simulink model "hybrid_aircraft"  (R2025b)
settings: Solver=ode4  StartTime=0.0  StopTime=1800  FixedStep=1  RelTol=1e-3
undefined symbols (not defined in the file): P_engine_max, P_motor_max
libraries: simulink x2

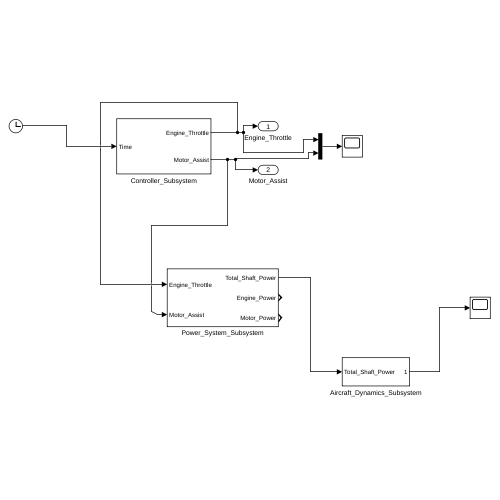
[thumbnail: Simulink's stored preview of the top-level diagram]
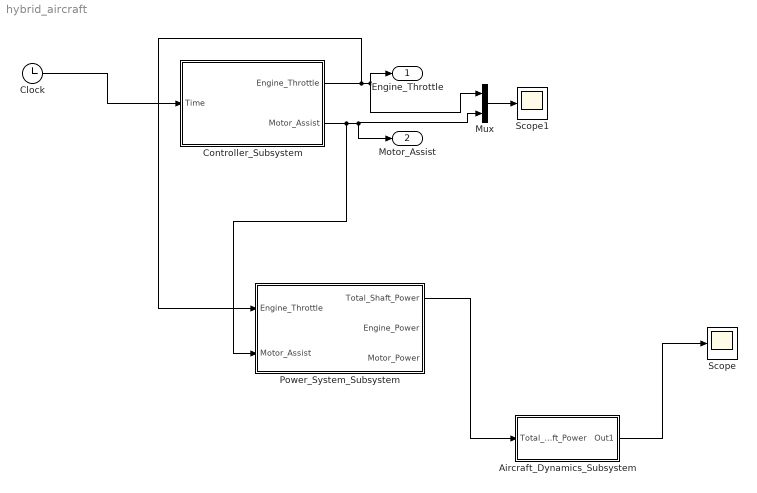
== system hybrid_aircraft ==
  Aircraft_Dynamics_Subsystem : Subsystem
  Clock : Clock
  Controller_Subsystem : Subsystem
  Mux : Mux  Inputs=2
  "Power_System_Subsystem " : Subsystem
  Scope : Scope
      settings: ActiveDisplayYMinimum=-317.16468253968424  ActiveDisplayYMaximum=2854.4821428571586
  Scope1 : Scope
      settings: ActiveDisplayYMinimum=-0.5175712749625333  ActiveDisplayYMaximum=1.2565171534864985
  Engine_Throttle : Outport
  Motor_Assist : Outport  Port=2
  wires:
  Clock/1 -> Controller_Subsystem/1(Time)
  Aircraft_Dynamics_Subsystem/1(Out1) -> Scope/1
  Controller_Subsystem/2(Motor_Assist) -> "Power_System_Subsystem "/2(Motor_Assist), Motor_Assist/1, Mux/2
  Controller_Subsystem/1(Engine_Throttle) -> "Power_System_Subsystem "/1(Engine_Throttle), Engine_Throttle/1, Mux/1
  Mux/1 -> Scope1/1
  "Power_System_Subsystem "/1(Total_Shaft_Power) -> Aircraft_Dynamics_Subsystem/1(Total_Shaft_Power)

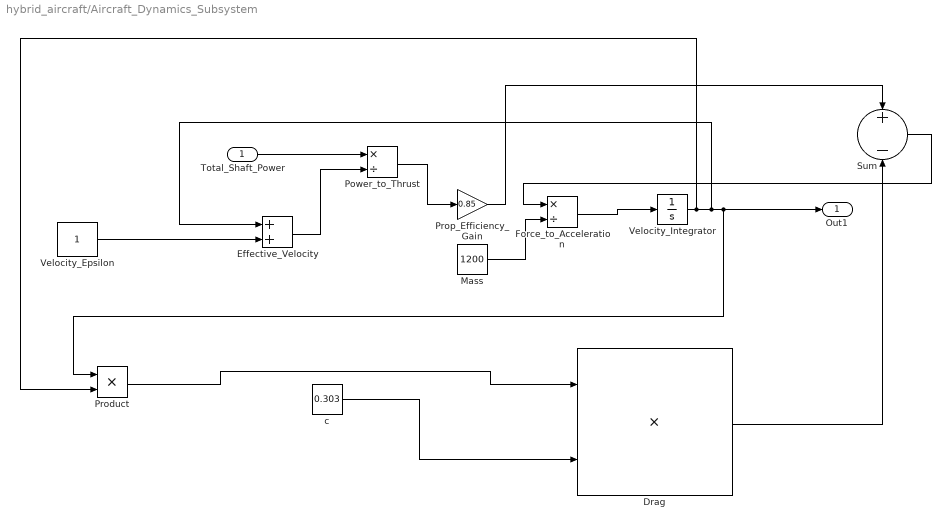
== system hybrid_aircraft/Aircraft_Dynamics_Subsystem ==
  Total_Shaft_Power : Inport
  Drag : Product
  Effective_Velocity : Sum
  Force_to_Acceleration : Product  Inputs=*/
  Mass : Constant  Value=1200
  Power_to_Thrust : Product  Inputs=*/
  Product : Product
  Prop_Efficiency_Gain : Gain  Gain=0.85
  Sum : Sum  Inputs=+-
  Velocity_Epsilon : Constant
  Velocity_Integrator : Integrator
  c : Constant  Value=0.303
  Out1 : Outport
  wires:
  Power_to_Thrust/1 -> Prop_Efficiency_Gain/1
  Mass/1 -> Force_to_Acceleration/2
  Total_Shaft_Power/1 -> Power_to_Thrust/1
  Force_to_Acceleration/1 -> Velocity_Integrator/1
  Velocity_Integrator/1 -> Product/2, Effective_Velocity/1, Product/1, Out1/1
  Effective_Velocity/1 -> Power_to_Thrust/2
  Velocity_Epsilon/1 -> Effective_Velocity/2
  Product/1 -> Drag/1
  c/1 -> Drag/2
  Drag/1 -> Sum/2
  Sum/1 -> Force_to_Acceleration/1
  Prop_Efficiency_Gain/1 -> Sum/1

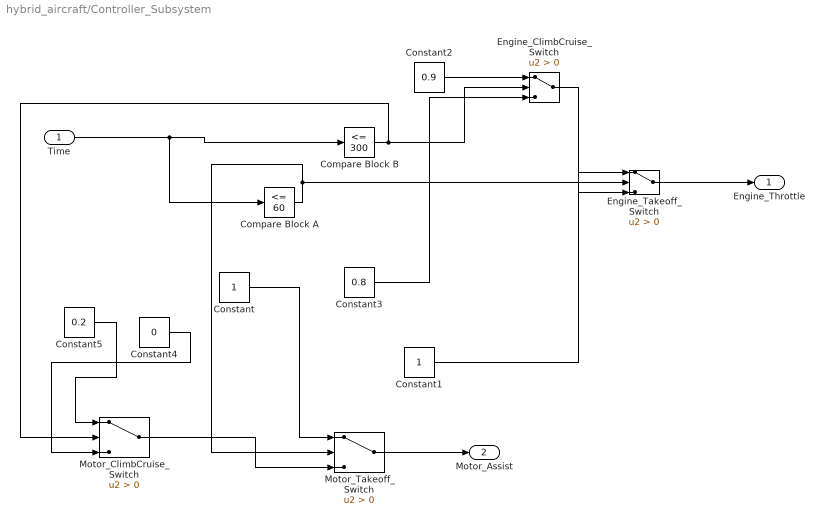
== system hybrid_aircraft/Controller_Subsystem ==
  Time : Inport
  Compare Block A : simulink/Logic and Bit Operations/Compare To Constant  relop=<=  const=60  OutDataTypeStr=boolean
  Compare Block B : simulink/Logic and Bit Operations/Compare To Constant  relop=<=  const=300  OutDataTypeStr=boolean
  Constant : Constant
  Constant1 : Constant
  Constant2 : Constant  Value=0.9
  Constant3 : Constant  Value=0.8
  Constant4 : Constant  Value=0
  Constant5 : Constant  Value=0.2
  Engine_ClimbCruise_Switch : Switch  Criteria=u2 > Threshold  SaturateOnIntegerOverflow=off  InputSameDT=off
  Engine_Takeoff_Switch : Switch  Criteria=u2 > Threshold  SaturateOnIntegerOverflow=off  InputSameDT=off
  Motor_ClimbCruise_Switch : Switch  Criteria=u2 > Threshold  SaturateOnIntegerOverflow=off  InputSameDT=off
  Motor_Takeoff_Switch : Switch  Criteria=u2 > Threshold  SaturateOnIntegerOverflow=off  InputSameDT=off
  Engine_Throttle : Outport
  Motor_Assist : Outport  Port=2
  wires:
  Time/1 -> Compare Block B/1, Compare Block A/1
  Constant2/1 -> Engine_ClimbCruise_Switch/1
  Constant3/1 -> Engine_ClimbCruise_Switch/3
  Constant1/1 -> Engine_Takeoff_Switch/1
  Engine_ClimbCruise_Switch/1 -> Engine_Takeoff_Switch/3
  Compare Block A/1 -> Motor_Takeoff_Switch/2, Engine_Takeoff_Switch/2
  Constant4/1 -> Motor_ClimbCruise_Switch/3
  Compare Block B/1 -> Motor_ClimbCruise_Switch/2, Engine_ClimbCruise_Switch/2
  Constant5/1 -> Motor_ClimbCruise_Switch/1
  Constant/1 -> Motor_Takeoff_Switch/1
  Motor_ClimbCruise_Switch/1 -> Motor_Takeoff_Switch/3
  Engine_Takeoff_Switch/1 -> Engine_Throttle/1
  Motor_Takeoff_Switch/1 -> Motor_Assist/1

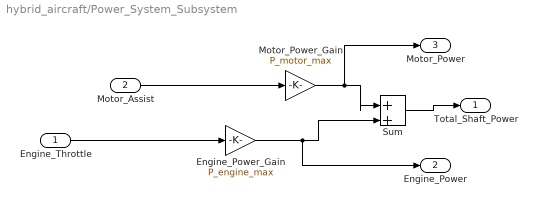
== system hybrid_aircraft/Power_System_Subsystem  ==
  Engine_Throttle : Inport
  Motor_Assist : Inport  Port=2
  Engine_Power_Gain : Gain  Gain=P_engine_max
  Motor_Power_Gain : Gain  Gain=P_motor_max
  Sum : Sum  Inputs=|++
  Total_Shaft_Power : Outport
  Engine_Power : Outport  Port=2
  Motor_Power : Outport  Port=3
  wires:
  Engine_Throttle/1 -> Engine_Power_Gain/1
  Motor_Assist/1 -> Motor_Power_Gain/1
  Motor_Power_Gain/1 -> Motor_Power/1, Sum/1
  Engine_Power_Gain/1 -> Engine_Power/1, Sum/2
  Sum/1 -> Total_Shaft_Power/1
